simulink model "yoyo2"  (R2013b)
settings: Solver=ode45  StartTime=0.0  StopTime=10.0  RelTol=1e-3
values from neighbouring files (symbols this model uses):
  A = 1    [yoyo_model.m]    (also in yoyo_model_simulate.m; yoyo_model_testing_lqi.m)
  B = phi    [yoyo_model.m]    (also in yoyo_model_simulate.m; yoyo_model_testing_lqi.m = 1)
  C = 1    [yoyo_model.m]    (also in yoyo_model_simulate.m; yoyo_model_testing_lqi.m)
  D = 0    [yoyo_model.m]    (also in yoyo_model_simulate.m; yoyo_model_testing_lqi.m)
  H = 1    [yoyo_model.m]    (also in yoyo_model_simulate.m = -100; yoyo_model_testing_lqi.m)
  K = 1    [yoyo_model.m]    (also in yoyo_model_simulate.m = 0.001; yoyo_model_testing_lqi.m)
  yr = 0    [yoyo_model.m]    (also in yoyo_model_simulate.m; yoyo_model_testing_lqi.m)
settings Model: Creator=thomasesch  LastModifiedBy=thomasesch

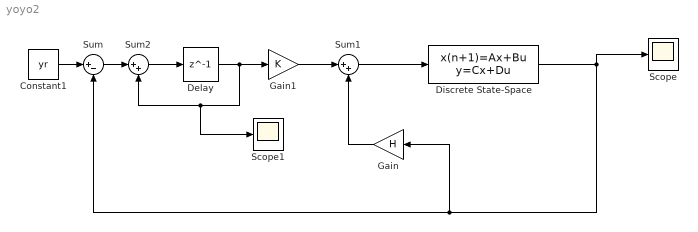
== system yoyo2 ==
  Constant1 : Constant  Value=yr
  Delay : Delay  DelayLength=1
  Discrete State-Space : DiscreteStateSpace  A=A  B=B  C=C  D=D
  Gain : Gain  Gain=H
  Gain1 : Gain  Gain=K
  Scope : Scope
  Scope1 : Scope
  Sum : Sum  Inputs=|+-
  Sum1 : Sum  Inputs=|++
  Sum2 : Sum  Inputs=|++
  wires:
  Discrete State-Space/1 -> Gain/1, Sum/2, Scope/1
  Sum1/1 -> Discrete State-Space/1
  Constant1/1 -> Sum/1
  Sum/1 -> Sum2/1
  Sum2/1 -> Delay/1
  Delay/1 -> Scope1/1, Sum2/2, Gain1/1
  Gain1/1 -> Sum1/1
  Gain/1 -> Sum1/2
